simulink model "PendulumInverseSIMU_theta"  (Simulink 10.0)
settings: Solver=ode45  StartTime=ti  StopTime=tf  FixedStep=0.001  RelTol=1e-3  EnableMultiTasking=on
undefined symbols (not defined in the file): g, gain, J, l, m, Mcart, n, Noise, theta
libraries: simulink x1
settings Model: Creator=huojiaxi  LastModifiedBy=huojiaxi  ExtModeTrigMode=oneshot  ExtModeArmWhenConnect=off
settings DataIOCC: SignalLoggingSaveFormat=ModelDataLogs
settings OptimizationCC: BooleanDataType=off  LifeSpan=auto
settings DebuggingCC: SaveWithParameterizedLinksMsg=none  SignalResolutionControl=TryResolveAllWithWarning  MultiTaskDSMMsg=warning  MultiTaskCondExecSysMsg=none  SFUnexpectedBacktrackingDiag=error  SFNoUnconditionalDefaultTransitionDiag=error  SFExecutionAtInitializationDiag=warning  ArithmeticOperatorsInVariantConditions=error
settings HardwareCC: ProdBitPerPointer=64  ProdBitPerSizeT=64  ProdBitPerPtrDiffT=64  ProdLargestAtomicFloat=Float  ProdIntDivRoundTo=Zero  ProdEndianess=LittleEndian  ProdWordSize=64  ProdHWDeviceType=Intel->x86-64 (Windows64)  TargetUnknown=on
settings SFSimCC: SimUseLocalCustomCode=on  CustomCodeUndefinedFunction=FilterOut
settings RTWCC: RTWUseLocalCustomCode=on
settings CodeAppCC: StateflowObjectComments=off
settings GRTTargetCC: TargetLangStandard=C99 (ISO)
settings ConfigComp: CovSaveCumulativeToWorkspaceVar=off  CovSaveSingleToWorkspaceVar=off

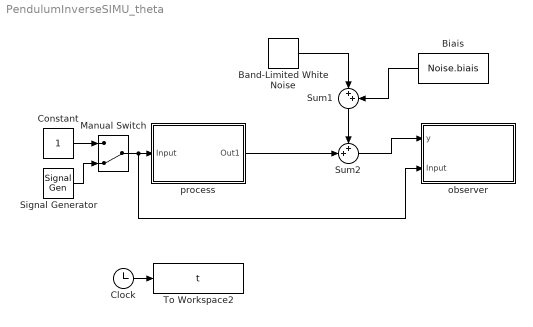
== system PendulumInverseSIMU_theta ==
  Band-Limited White Noise : simulink/Sources/Band-Limited White Noise  Cov=Noise.power  Ts=Noise.sampling  seed=Noise.seed
  Biais : Constant  Value=Noise.biais
  Clock : Clock
  Constant : Constant
  Manual Switch : ManualSwitch  CurrentSetting=0
  Signal Generator : SignalGenerator  Units=rad/sec
  Sum1 : Sum  Inputs=|++
  Sum2 : Sum  Inputs=++|
  To Workspace2 : ToWorkspace  VariableName=t  SampleTime=-1
  observer : Subsystem
  process : Subsystem
  wires:
  Sum1/1 -> Sum2/1
  Biais/1 -> Sum1/2
  Band-Limited White Noise/1 -> Sum1/1
  Sum2/1 -> observer/1(y)
  process/1(Out1) -> Sum2/2
  Clock/1 -> To Workspace2/1
  Manual Switch/1 -> observer/2(Input), process/1(Input)
  Constant/1 -> Manual Switch/1
  Signal Generator/1 -> Manual Switch/2

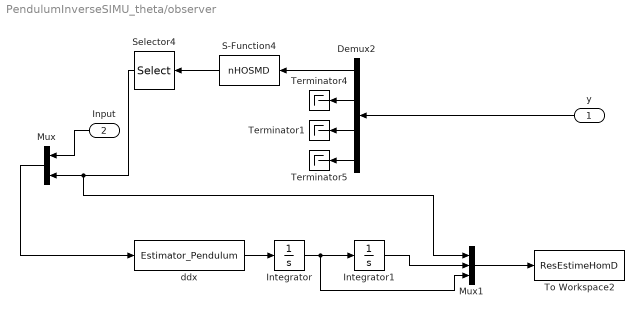
== system PendulumInverseSIMU_theta/observer ==
  y : Inport
  Input : Inport  Port=2
  Demux2 : Demux
  Integrator : Integrator
  Integrator1 : Integrator
  Mux : Mux  Inputs=2
  Mux1 : Mux  Inputs=3
  S-Function4 : S-Function  FunctionName=nHOSMD  Parameters=n,gain,theta  SFunctionDeploymentMode=off  EnableBusSupport=off
  Selector4 : Selector  InputPortWidth=n+1  IndexOptions=Index vector (dialog)  Indices=[1 2]  OutputSizes=1
  Terminator1 : Terminator
  Terminator4 : Terminator
  Terminator5 : Terminator
  To Workspace2 : ToWorkspace  VariableName=ResEstimeHomD  SampleTime=-1
  ddx : S-Function  FunctionName=Estimator_Pendulum  Parameters=Mcart,m,l,g,J  SFunctionDeploymentMode=off  EnableBusSupport=off
  wires:
  Demux2/3 -> Terminator1/1
  Demux2/2 -> Terminator4/1
  Demux2/1 -> S-Function4/1
  S-Function4/1 -> Selector4/1
  Demux2/4 -> Terminator5/1
  y/1 -> Demux2/1
  Selector4/1 -> Mux1/1, Mux/2
  ddx/1 -> Integrator/1
  Integrator/1 -> Mux1/3, Integrator1/1
  Mux1/1 -> To Workspace2/1
  Input/1 -> Mux/1
  Mux/1 -> ddx/1
  Integrator1/1 -> Mux1/2

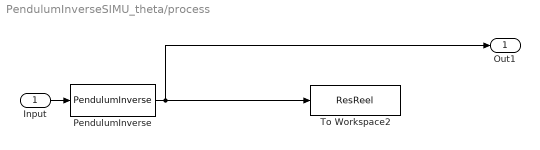
== system PendulumInverseSIMU_theta/process ==
  Input : Inport
  PendulumInverse : S-Function  FunctionName=PendulumInverse  Parameters=Mcart,m,l,g,J  SFunctionDeploymentMode=off  EnableBusSupport=off
  To Workspace2 : ToWorkspace  VariableName=ResReel  SampleTime=-1
  Out1 : Outport
  wires:
  Input/1 -> PendulumInverse/1
  PendulumInverse/1 -> To Workspace2/1, Out1/1
